simulink library "environmental_module"  (R2025b)
settings: Solver=VariableStepAuto  StartTime=0.0  StopTime=10.0  RelTol=1e-3
settings Model: Creator=ciepm  LastModifiedBy=charlielenk

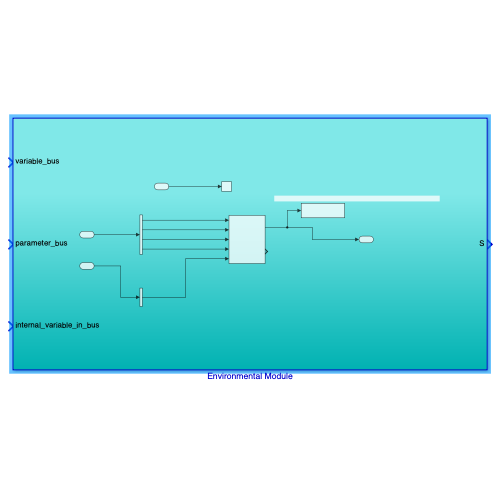
[thumbnail: Simulink's stored preview of the top-level diagram]
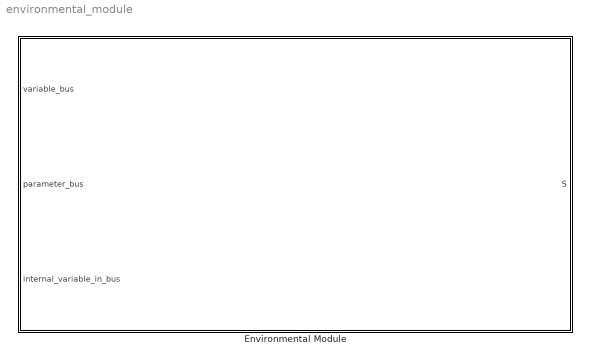
== system environmental_module ==
  Environmental Module : Subsystem

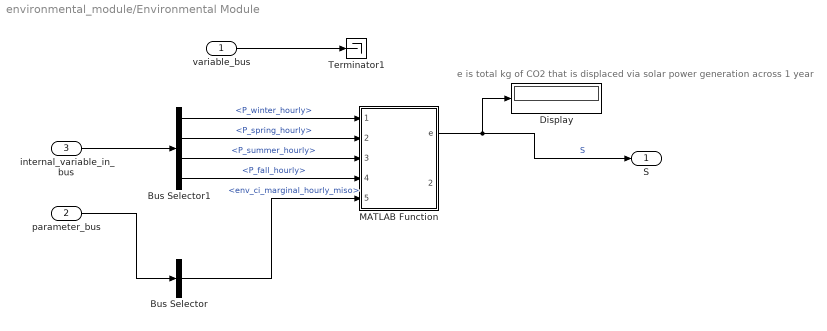
== system environmental_module/Environmental Module ==
  note: e is total kg of CO2 that is displaced via solar power generation across 1 year
  variable_bus : Inport
  parameter_bus : Inport  Port=2
  internal_variable_in_bus : Inport  Port=3
  Bus Selector : BusSelector  OutputSignals=env_ci_marginal_hourly_miso
  Bus Selector1 : BusSelector  OutputSignals=P_winter_hourly,P_spring_hourly,P_summer_hourly,P_fall_hourly
  Display : Display
  MATLAB Function : MATLAB Function  TreatAsAtomicUnit=on
  Terminator1 : Terminator
  S : Outport
  wires:
  Bus Selector1/4 -> MATLAB Function/4(P_hourly_Fa)  "<P_fall_hourly>"
  Bus Selector1/3 -> MATLAB Function/3(P_hourly_Su)  "<P_summer_hourly>"
  Bus Selector1/2 -> MATLAB Function/2(P_hourly_Sp)  "<P_spring_hourly>"
  Bus Selector1/1 -> MATLAB Function/1(P_hourly_Wi)  "<P_winter_hourly>"
  internal_variable_in_bus/1 -> Bus Selector1/1
  parameter_bus/1 -> Bus Selector/1
  variable_bus/1 -> Terminator1/1
  Bus Selector/1 -> MATLAB Function/5(CI_hourly)  "<env_ci_marginal_hourly_miso>"
  MATLAB Function/1(e) -> Display/1, S/1  "S"

== matlab function environmental_module/Environmental Module/MATLAB Function ==
  data: P_hourly_Wi input; P_hourly_Sp input; P_hourly_Su input; P_hourly_Fa input; e output; CI_hourly input; P_hourly output
function [e, P_hourly] = fcn(P_hourly_Wi,P_hourly_Sp,P_hourly_Su,P_hourly_Fa, CI_hourly)
% CI hourly should just be 96 vals long--> get representative 24 hour
% values for each of the 4 seasons, starting with winter
P_hourly = [P_hourly_Wi; P_hourly_Sp; P_hourly_Su; P_hourly_Fa];
disp(P_hourly);
E_MWh = P_hourly / 1e6;      % assuming P_hourly is in W-->converting to MWh for each hour
co2_displaced_hourly_lbs = E_MWh .* CI_hourly; % in units of lbs CO2e--> CI_hourly is in lbs CO2/MWh
co2_displaced_hourly_kgs = co2_displaced_hourly_lbs / 2.205;
% disp(E_MWh*1000); %displaying kWh produced each hour
%E_Daily_MWh = sum(E_MWh);
%disp('Energy Production (MWh) for the day:')
%disp(E_Daily_MWh)
e = sum(co2_displaced_hourly_kgs)*91.25; % kg CO2eq displaced from marginal MISO emissions--> FOR 1 YEAR
%disp('kg CO2 emissions for the year:')
%disp(e)



end
